simulink model "ScriptDemo"  (R2022b)
settings: configuration reference "TmVcThermal_Configuration_sub" (kept outside this file)
undefined symbols (not defined in the file): aaaa, bbbb, cTmComprCtrl_D_u8HvacFlowTable_db, cTmComprCtrl_D_u8HvacFlowTable_sw, cTmComprCtrl_n_i16ChillCmpIMax, cTmComprCtrl_n_i16ChillCmpIMin, cTmComprCtrl_n_i16ChillCmpIMin666, cTmComprCtrl_n_i16ChillCmpPMax, cTmComprCtrl_n_i16ChillCmpPMin, cTmComprCtrl_n_i16CmpChillCoolRpmKiMax, cTmComprCtrl_n_i16CmpChillCoolRpmKiMin, cTmComprCtrl_n_i16CmpChillCoolRpmKpMax, cTmComprCtrl_n_i16CmpChillCoolRpmKpMin, cTmComprCtrl_n_i16CmpCoolRpmKiMax, cTmComprCtrl_n_i16CmpCoolRpmKiMin, cTmComprCtrl_n_i16CmpCoolRpmKpMax, cTmComprCtrl_n_i16CmpCoolRpmKpMin, cTmComprCtrl_n_i16SM4CmpHeatKiMax, cTmComprCtrl_n_i16SM4CmpHeatKiMin, cTmComprCtrl_n_i16SM4CmpHeatKpMax, cTmComprCtrl_n_i16SM4CmpHeatKpMin, cTmComprCtrl_n_i16SM5CmpHeatKiMax, cTmComprCtrl_n_i16SM5CmpHeatKiMin, cTmComprCtrl_n_i16SM5CmpHeatKpMax, cTmComprCtrl_n_i16SM5CmpHeatKpMin, cTmComprCtrl_n_i16SM6CmpHeatKiMax, cTmComprCtrl_n_i16SM6CmpHeatKiMin, cTmComprCtrl_n_i16SM6CmpHeatKpMax, cTmComprCtrl_n_i16SM6CmpHeatKpMin, cTmComprCtrl_n_u16CmpMaxSpdFanFltLimt, cTmComprCtrl_n_u16CmpMaxSpdLoSidePFltLimt, cTmComprCtrl_n_u16CmpMaxSpdSensorFltLimt, cTmComprCtrl_n_u16CompMinRpm, cTmComprCtrl_n_u16CompRpmIncThres, cTmComprCtrl_t_u16BattCooltFFPeriod, cTmComprCtrl_t_u16BattCooltPIPeriod, cTmComprCtrl_t_u16CmpCoolFFPeriod, cTmComprCtrl_t_u16CmpCoolPIPeriod, cTmComprCtrl_t_u16CoolCmpChillFFPeriod, cTmComprCtrl_t_u16CoolCmpChillPIPeriod, cTmComprCtrl_t_u16SM4CmpHeatFFPeriod, cTmComprCtrl_t_u16SM4CmpHeatPIPeriod, cTmComprCtrl_t_u16SM5CmpHeatFFPeriod, cTmComprCtrl_t_u16SM5CmpHeatPIPeriod, cTmComprCtrl_t_u16SM6CmpHeatFFPeriod, cTmComprCtrl_t_u16SM6CmpHeatPIPeriod, cTmComprCtrl_Te_EvapClearInteg, cTmComprCtrl_Te_i16HpReqTempSaturoffset, cTmComprCtrl_Te_i16SatLpReplaceDiff, cTmComprCtrl_Te_i16SM3BatDiffStartEvapDecOffset, cTmComprCtrl_Te_i16SM3EvapLo, cTmComprCtrl_Te_i16SM3TBatDiffEntEvapDecOffset, cTmComprCtrl_Te_i16SM3TBatDiffEntEvapDecOffsetQuit, cTmComprCtrl_Te_s32ErrCmpChillPIContinueCoolH, cTmComprCtrl_Te_s32ErrCmpChillPIContinueCoolL, cTmComprCtrl_Te_s32ErrCmpPIContinueChillH, cTmComprCtrl_Te_s32ErrCmpPIContinueChillL, cTmComprCtrl_Te_s32ErrCmpPIContinueCoolH, cTmComprCtrl_Te_s32ErrCmpPIContinueCoolL, cTmComprCtrl_Te_s32ErrCmpPIContinueHeatH ... (+398)
libraries: simulink x782, PCMULib x640, simulink_need_slupdate x4
(part 23 of 41)

== system ScriptDemo/Create/createMerge/Before/SM5/SM5_Ki ==
  sTmComprCtrl_D_u8HvacFlowLevel : Inport  OutDataTypeStr=uint8
  sTmSigProces_Te_s32SatLp : Inport  Port=2
  rTmComprCtrl_Te_s32TempError : Inport  Port=3
  Data Type Conversion : DataTypeConversion  OutDataTypeStr=uint16  SaturateOnIntegerOverflow=off  RndMeth=Floor
  Flow2Rpm : Subsystem  mask{BlwHeatLevel_db=cTmComprCtrl_D_u8HvacFlowTable_db, BlwHeatLevel_sw=cTmComprCtrl_D_u8HvacFlowTable_sw, FFBlw1=mTmComprCtrl_n_u16KiSM5CompHeatRpm_Flow1, FFBlw1_Y=mTmComprCtrl_n_u16KiSM5CompHeatRpm_Flow1_Y, FFBlw1_X=mTmComprCtrl_n_u16KiSM5CompHeatRpm_Flow1_X, FFBlw3=mTmComprCtrl_n_u16KiSM5CompHeatRpm_Flow3, FFBlw3_Y=mTmComprCtrl_n_u16KiSM5CompHeatRpm_Flow3_Y, FFBlw3_X=mTmComprCtrl_n_u16KiSM5CompHeatRpm_Flow3_X, FFBlw5=mTmComprCtrl_n_u16KiSM5CompHeatRpm_Flow5, FFBlw5_Y=mTmComprCtrl_n_u16KiSM5CompHeatRpm_Flow5_Y, FFBlw5_X=mTmComprCtrl_n_u16KiSM5CompHeatRpm_Flow5_X, FFBlw7=mTmComprCtrl_n_u16KiSM5CompHeatRpm_Flow7, FFBlw7_Y=mTmComprCtrl_n_u16KiSM5CompHeatRpm_Flow7_Y, FFBlw7_X=mTmComprCtrl_n_u16KiSM5CompHeatRpm_Flow7_X, FFBlw9=mTmComprCtrl_n_u16KiSM5CompHeatRpm_Flow9, FFBlw9_Y=mTmComprCtrl_n_u16KiSM5CompHeatRpm_Flow9_Y, FFBlw9_X=mTmComprCtrl_n_u16KiSM5CompHeatRpm_Flow9_X}
      mask DialogControl ParameterGroupVar Prompt: 参数
  SM5Ki : Outport
  wires:
  Flow2Rpm/1(Flow2Rpm) -> Data Type Conversion/1
  Data Type Conversion/1 -> SM5Ki/1
  sTmComprCtrl_D_u8HvacFlowLevel/1 -> Flow2Rpm/1(md_u8Blw)
  sTmSigProces_Te_s32SatLp/1 -> Flow2Rpm/2(breakpoint1)
  rTmComprCtrl_Te_s32TempError/1 -> Flow2Rpm/3(breakpoint2)

== system ScriptDemo/Create/createMerge/Before/SM5/SM5_Kp ==
  sTmComprCtrl_D_u8HvacFlowLevel : Inport  OutDataTypeStr=uint8
  sTmSigProces_Te_s32SatLp : Inport  Port=2
  rTmComprCtrl_Te_s32TempError : Inport  Port=3
  Data Type Conversion : DataTypeConversion  OutDataTypeStr=uint16  SaturateOnIntegerOverflow=off  RndMeth=Floor
  Flow2Rpm : Subsystem  mask{BlwHeatLevel_db=cTmComprCtrl_D_u8HvacFlowTable_db, BlwHeatLevel_sw=cTmComprCtrl_D_u8HvacFlowTable_sw, FFBlw1=mTmComprCtrl_n_u16KpSM5CompHeatRpm_Flow1, FFBlw1_Y=mTmComprCtrl_n_u16KpSM5CompHeatRpm_Flow1_Y, FFBlw1_X=mTmComprCtrl_n_u16KpSM5CompHeatRpm_Flow1_X, FFBlw3=mTmComprCtrl_n_u16KpSM5CompHeatRpm_Flow3, FFBlw3_Y=mTmComprCtrl_n_u16KpSM5CompHeatRpm_Flow3_Y, FFBlw3_X=mTmComprCtrl_n_u16KpSM5CompHeatRpm_Flow3_X, FFBlw5=mTmComprCtrl_n_u16KpSM5CompHeatRpm_Flow5, FFBlw5_Y=mTmComprCtrl_n_u16KpSM5CompHeatRpm_Flow5_Y, FFBlw5_X=mTmComprCtrl_n_u16KpSM5CompHeatRpm_Flow5_X, FFBlw7=mTmComprCtrl_n_u16KpSM5CompHeatRpm_Flow7, FFBlw7_Y=mTmComprCtrl_n_u16KpSM5CompHeatRpm_Flow7_Y, FFBlw7_X=mTmComprCtrl_n_u16KpSM5CompHeatRpm_Flow7_X, FFBlw9=mTmComprCtrl_n_u16KpSM5CompHeatRpm_Flow9, FFBlw9_Y=mTmComprCtrl_n_u16KpSM5CompHeatRpm_Flow9_Y, FFBlw9_X=mTmComprCtrl_n_u16KpSM5CompHeatRpm_Flow9_X}
      mask DialogControl ParameterGroupVar Prompt: 参数
  SM5Kp : Outport
  wires:
  Flow2Rpm/1(Flow2Rpm) -> Data Type Conversion/1
  Data Type Conversion/1 -> SM5Kp/1
  sTmSigProces_Te_s32SatLp/1 -> Flow2Rpm/2(breakpoint1)
  rTmComprCtrl_Te_s32TempError/1 -> Flow2Rpm/3(breakpoint2)
  sTmComprCtrl_D_u8HvacFlowLevel/1 -> Flow2Rpm/1(md_u8Blw)

== system ScriptDemo/Create/createMerge/Before/SM6/ID26282_SM6FF ==
  note: TODO: 这里需要确认下需求
  sTmComprCtrl_D_u8HvacFlowLevel : Inport  OutDataTypeStr=uint8
  sTmSigProces_Te_s32TempInlet : Inport  Port=2
  sTmSigProces_Te_s32HeatrAirTReqRamp : Inport  Port=3
  Enable : EnablePort
  Flow2Rpm : Subsystem  mask{BlwHeatLevel_db=cTmComprCtrl_D_u8HvacFlowTable_db, BlwHeatLevel_sw=cTmComprCtrl_D_u8HvacFlowTable_sw, FFBlw1=mTmComprCtrl_n_u16FFSM6CompHeatRpm_Flow1, FFBlw1_Y=mTmComprCtrl_n_u16FFSM6CompHeatRpm_Flow1_Y, FFBlw1_X=mTmComprCtrl_n_u16FFSM6CompHeatRpm_Flow1_X, FFBlw3=mTmComprCtrl_n_u16FFSM6CompHeatRpm_Flow3, FFBlw3_Y=mTmComprCtrl_n_u16FFSM6CompHeatRpm_Flow3_Y, FFBlw3_X=mTmComprCtrl_n_u16FFSM6CompHeatRpm_Flow3_X, FFBlw5=mTmComprCtrl_n_u16FFSM6CompHeatRpm_Flow5, FFBlw5_Y=mTmComprCtrl_n_u16FFSM6CompHeatRpm_Flow5_Y, FFBlw5_X=mTmComprCtrl_n_u16FFSM6CompHeatRpm_Flow5_X, FFBlw7=mTmComprCtrl_n_u16FFSM6CompHeatRpm_Flow7, FFBlw7_Y=mTmComprCtrl_n_u16FFSM6CompHeatRpm_Flow7_Y, FFBlw7_X=mTmComprCtrl_n_u16FFSM6CompHeatRpm_Flow7_X, FFBlw9=mTmComprCtrl_n_u16FFSM6CompHeatRpm_Flow9, FFBlw9_Y=mTmComprCtrl_n_u16FFSM6CompHeatRpm_Flow9_Y, FFBlw9_X=mTmComprCtrl_n_u16FFSM6CompHeatRpm_Flow9_X}
      mask DialogControl ParameterGroupVar Prompt: 参数
  SM6FF : Outport
  wires:
  Flow2Rpm/1(Flow2Rpm) -> SM6FF/1
  sTmComprCtrl_D_u8HvacFlowLevel/1 -> Flow2Rpm/1(md_u8Blw)
  sTmSigProces_Te_s32HeatrAirTReqRamp/1 -> Flow2Rpm/3(breakpoint2)
  sTmSigProces_Te_s32TempInlet/1 -> Flow2Rpm/2(breakpoint1)

== system ScriptDemo/Create/createMerge/Before/SM6/ID26284_SM6Error ==
  note: 暖风芯体背风温度目标值∈[0, 80] ℃ 。
  note: 无PTC补热
  note: PTC 补热模式
  sTmSigProces_Te_s32SatHp : Inport
  yTmHvchCtrl_B_HpcPtcEnad : Inport  Port=2
  sTmSigProces_Te_s32HeatrAirTReqRamp : Inport  Port=3
  sTmSigProces_Te_s32HvacHexAirTFilter : Inport  Port=4
  Add2 : Sum
  Constant5 : Constant  Value=cTmComprCtrl_Te_i16HpReqTempSaturoffset
  NegAndPosCheck 4 : Subsystem  AncestorBlock=CustomLib/TempNegAndPosCheck
  NegAndPosCheck 5 : Subsystem  AncestorBlock=CustomLib/TempNegAndPosCheck
  Saturation2 : Saturate  UpperLimit=70  LowerLimit=15
  Switch2 : Switch  Criteria=u2 ~= 0  SaturateOnIntegerOverflow=off  InputSameDT=off
  Terminator : Terminator
  Terminator1 : Terminator
  Unary Minus : UnaryMinus
  rTmComprCtrl_Te_s32TempError : Outport
  wires:
  sTmSigProces_Te_s32SatHp/1 -> NegAndPosCheck 4/2(Acture)
  NegAndPosCheck 5/1(Dvt) -> Switch2/3
  sTmSigProces_Te_s32HeatrAirTReqRamp/1 -> Saturation2/1
  Switch2/1 -> Unary Minus/1
  NegAndPosCheck 5/2(Dvt_PosFlag) -> Terminator/1
  NegAndPosCheck 4/1(Dvt) -> Switch2/1
  Constant5/1 -> Add2/1
  NegAndPosCheck 4/2(Dvt_PosFlag) -> Terminator1/1
  sTmSigProces_Te_s32HvacHexAirTFilter/1 -> NegAndPosCheck 5/2(Acture)
  yTmHvchCtrl_B_HpcPtcEnad/1 -> Switch2/2
  Saturation2/1 -> NegAndPosCheck 5/1(SetPoint), Add2/2
  Add2/1 -> NegAndPosCheck 4/1(SetPoint)
  Unary Minus/1 -> rTmComprCtrl_Te_s32TempError/1

== system ScriptDemo/Create/createMerge/Before/SM6/SM6FFEnable ==
  xTmComprCtrl_B_CompOnReqCompOn : Inport  OutDataTypeStr=boolean
  Compare To Constant2 : simulink/Logic and Bit Operations/Compare To Constant  relop===  const=0  OutDataTypeStr=boolean
  Compare To Constant3 : simulink/Logic and Bit Operations/Compare To Constant  relop===  const=1  OutDataTypeStr=boolean
  Logical Operator3 : Logic  AllPortsSameDT=off  OutDataTypeStr=boolean
  PeriodTrig : Subsystem  mask{CounterLim=cTmComprCtrl_t_u16SM6CmpHeatFFPeriod}
      mask DialogControl ParameterGroupVar Prompt: 参数
  Unit Delay : UnitDelay  SampleTime=-1  HasFrameUpgradeWarning=on
  SM6FFEnable_B_SM6FFEnable : Outport  OutDataTypeStr=boolean
  wires:
  Unit Delay/1 -> Compare To Constant2/1
  [xTmComprCtrl_B_CompOnReqCompOn] -> Compare To Constant3/1, Unit Delay/1
  Compare To Constant2/1 -> Logical Operator3/1
  Logical Operator3/1 -> PeriodTrig/1(Counter_Reset)
  Compare To Constant3/1 -> Logical Operator3/2
  xTmComprCtrl_B_CompOnReqCompOn/1 -> [xTmComprCtrl_B_CompOnReqCompOn]
  PeriodTrig/1(Counter_Trig) -> SM6FFEnable_B_SM6FFEnable/1

== system ScriptDemo/Create/createMerge/Before/SM6/SM6_Ki ==
  sTmComprCtrl_D_u8HvacFlowLevel : Inport  OutDataTypeStr=uint8
  sTmSigProces_Te_s32TempInlet : Inport  Port=2
  rTmComprCtrl_Te_s32TempError : Inport  Port=3
  Flow2Rpm : Subsystem  mask{BlwHeatLevel_db=cTmComprCtrl_D_u8HvacFlowTable_db, BlwHeatLevel_sw=cTmComprCtrl_D_u8HvacFlowTable_sw, FFBlw1=mTmComprCtrl_n_u16KiSM6CompHeatRpm_Flow1, FFBlw1_Y=mTmComprCtrl_n_u16KiSM6CompHeatRpm_Flow1_Y, FFBlw1_X=mTmComprCtrl_n_u16KiSM6CompHeatRpm_Flow1_X, FFBlw3=mTmComprCtrl_n_u16KiSM6CompHeatRpm_Flow3, FFBlw3_Y=mTmComprCtrl_n_u16KiSM6CompHeatRpm_Flow3_Y, FFBlw3_X=mTmComprCtrl_n_u16KiSM6CompHeatRpm_Flow3_X, FFBlw5=mTmComprCtrl_n_u16KiSM6CompHeatRpm_Flow5, FFBlw5_Y=mTmComprCtrl_n_u16KiSM6CompHeatRpm_Flow5_Y, FFBlw5_X=mTmComprCtrl_n_u16KiSM6CompHeatRpm_Flow5_X, FFBlw7=mTmComprCtrl_n_u16KiSM6CompHeatRpm_Flow7, FFBlw7_Y=mTmComprCtrl_n_u16KiSM6CompHeatRpm_Flow7_Y, FFBlw7_X=mTmComprCtrl_n_u16KiSM6CompHeatRpm_Flow7_X, FFBlw9=mTmComprCtrl_n_u16KiSM6CompHeatRpm_Flow9, FFBlw9_Y=mTmComprCtrl_n_u16KiSM6CompHeatRpm_Flow9_Y, FFBlw9_X=mTmComprCtrl_n_u16KiSM6CompHeatRpm_Flow9_X}
      mask DialogControl ParameterGroupVar Prompt: 参数
  SM6Ki : Outport
  wires:
  Flow2Rpm/1(Flow2Rpm) -> SM6Ki/1
  sTmSigProces_Te_s32TempInlet/1 -> Flow2Rpm/2(breakpoint1)
  sTmComprCtrl_D_u8HvacFlowLevel/1 -> Flow2Rpm/1(md_u8Blw)
  rTmComprCtrl_Te_s32TempError/1 -> Flow2Rpm/3(breakpoint2)

== system ScriptDemo/Create/createMerge/Before/SM6/SM6_Kp ==
  sTmComprCtrl_D_u8HvacFlowLevel : Inport  OutDataTypeStr=uint8
  sTmSigProces_Te_s32TempInlet : Inport  Port=2
  rTmComprCtrl_Te_s32TempError : Inport  Port=3
  Flow2Rpm : Subsystem  mask{BlwHeatLevel_db=cTmComprCtrl_D_u8HvacFlowTable_db, BlwHeatLevel_sw=cTmComprCtrl_D_u8HvacFlowTable_sw, FFBlw1=mTmComprCtrl_n_u16KpSM6CompHeatRpm_Flow1, FFBlw1_Y=mTmComprCtrl_n_u16KpSM6CompHeatRpm_Flow1_Y, FFBlw1_X=mTmComprCtrl_n_u16KpSM6CompHeatRpm_Flow1_X, FFBlw3=mTmComprCtrl_n_u16KpSM6CompHeatRpm_Flow3, FFBlw3_Y=mTmComprCtrl_n_u16KpSM6CompHeatRpm_Flow3_Y, FFBlw3_X=mTmComprCtrl_n_u16KpSM6CompHeatRpm_Flow3_X, FFBlw5=mTmComprCtrl_n_u16KpSM6CompHeatRpm_Flow5, FFBlw5_Y=mTmComprCtrl_n_u16KpSM6CompHeatRpm_Flow5_Y, FFBlw5_X=mTmComprCtrl_n_u16KpSM6CompHeatRpm_Flow5_X, FFBlw7=mTmComprCtrl_n_u16KpSM6CompHeatRpm_Flow7, FFBlw7_Y=mTmComprCtrl_n_u16KpSM6CompHeatRpm_Flow7_Y, FFBlw7_X=mTmComprCtrl_n_u16KpSM6CompHeatRpm_Flow7_X, FFBlw9=mTmComprCtrl_n_u16KpSM6CompHeatRpm_Flow9, FFBlw9_Y=mTmComprCtrl_n_u16KpSM6CompHeatRpm_Flow9_Y, FFBlw9_X=mTmComprCtrl_n_u16KpSM6CompHeatRpm_Flow9_X}
      mask DialogControl ParameterGroupVar Prompt: 参数
  SM6Kp : Outport
  wires:
  Flow2Rpm/1(Flow2Rpm) -> SM6Kp/1
  sTmComprCtrl_D_u8HvacFlowLevel/1 -> Flow2Rpm/1(md_u8Blw)
  sTmSigProces_Te_s32TempInlet/1 -> Flow2Rpm/2(breakpoint1)
  rTmComprCtrl_Te_s32TempError/1 -> Flow2Rpm/3(breakpoint2)

== system ScriptDemo/Create/createPorts/createPortsGotoUpdate/After/AllowedPower ==
  note: 压缩机不满足开启条件
  note: 压缩机满足开启条件
  note: 压缩机允许功率
  sTmIn_Pw_s32HvCoolgAllwd : Inport
  xTmComprCtrl_B_CompOnReqCompOn : Inport  Port=2
  Compare To Constant : simulink/Logic and Bit Operations/Compare To Constant  relop=>=  const=6500  OutDataTypeStr=boolean
  Compare To Constant1 : simulink/Logic and Bit Operations/Compare To Constant  relop===  const=6500  OutDataTypeStr=boolean
  Constant2 : Constant  Value=0  OutDataTypeStr=single
  Constant4 : Constant  Value=6500  OutDataTypeStr=single
  Switch1 : Switch  Criteria=u2 ~= 0  SaturateOnIntegerOverflow=off  InputSameDT=off
  Switch3 : Switch  Criteria=u2 ~= 0  Threshold=6500  SaturateOnIntegerOverflow=off  InputSameDT=off
  sTmComprCtrl_Pw_s32ElacCmprMaxState : Outport
  yTmComprCtrl_B_HpcCoolgLimd : Outport  Port=2
  wires:
  sTmIn_Pw_s32HvCoolgAllwd/1 -> Switch3/3, Compare To Constant/1
  Constant2/1 -> Switch1/3
  xTmComprCtrl_B_CompOnReqCompOn/1 -> Switch1/2
  Switch3/1 -> Switch1/1
  Switch1/1 -> Compare To Constant1/1, sTmComprCtrl_Pw_s32ElacCmprMaxState/1
  Constant4/1 -> Switch3/1
  Compare To Constant/1 -> Switch3/2
  Compare To Constant1/1 -> yTmComprCtrl_B_HpcCoolgLimd/1

== system ScriptDemo/Create/createPorts/createPortsGotoUpdate/After1/AllowedPower ==
  note: 压缩机不满足开启条件
  note: 压缩机满足开启条件
  note: 压缩机允许功率
  sTmIn_Pw_s32HvCoolgAllwd : Inport
  xTmComprCtrl_B_CompOnReqCompOn : Inport  Port=2
  Compare To Constant : simulink/Logic and Bit Operations/Compare To Constant  relop=>=  const=6500  OutDataTypeStr=boolean
  Compare To Constant1 : simulink/Logic and Bit Operations/Compare To Constant  relop===  const=6500  OutDataTypeStr=boolean
  Constant2 : Constant  Value=0  OutDataTypeStr=single
  Constant4 : Constant  Value=6500  OutDataTypeStr=single
  Switch1 : Switch  Criteria=u2 ~= 0  SaturateOnIntegerOverflow=off  InputSameDT=off
  Switch3 : Switch  Criteria=u2 ~= 0  Threshold=6500  SaturateOnIntegerOverflow=off  InputSameDT=off
  sTmComprCtrl_Pw_s32ElacCmprMaxState : Outport
  yTmComprCtrl_B_HpcCoolgLimd : Outport  Port=2
  wires:
  sTmIn_Pw_s32HvCoolgAllwd/1 -> Switch3/3, Compare To Constant/1
  Constant2/1 -> Switch1/3
  xTmComprCtrl_B_CompOnReqCompOn/1 -> Switch1/2
  Switch3/1 -> Switch1/1
  Switch1/1 -> Compare To Constant1/1, sTmComprCtrl_Pw_s32ElacCmprMaxState/1
  Constant4/1 -> Switch3/1
  Compare To Constant/1 -> Switch3/2
  Compare To Constant1/1 -> yTmComprCtrl_B_HpcCoolgLimd/1

== system ScriptDemo/Create/createPorts/createPortsGotoUpdate/Before/AllowedPower ==
  note: 压缩机不满足开启条件
  note: 压缩机满足开启条件
  note: 压缩机允许功率
  sTmIn_Pw_s32HvCoolgAllwd : Inport
  xTmComprCtrl_B_CompOnReqCompOn : Inport  Port=2
  Compare To Constant : simulink/Logic and Bit Operations/Compare To Constant  relop=>=  const=6500  OutDataTypeStr=boolean
  Compare To Constant1 : simulink/Logic and Bit Operations/Compare To Constant  relop===  const=6500  OutDataTypeStr=boolean
  Constant2 : Constant  Value=0  OutDataTypeStr=single
  Constant4 : Constant  Value=6500  OutDataTypeStr=single
  Switch1 : Switch  Criteria=u2 ~= 0  SaturateOnIntegerOverflow=off  InputSameDT=off
  Switch3 : Switch  Criteria=u2 ~= 0  Threshold=6500  SaturateOnIntegerOverflow=off  InputSameDT=off
  sTmComprCtrl_Pw_s32ElacCmprMaxState : Outport
  yTmComprCtrl_B_HpcCoolgLimd : Outport  Port=2
  wires:
  sTmIn_Pw_s32HvCoolgAllwd/1 -> Switch3/3, Compare To Constant/1
  Constant2/1 -> Switch1/3
  xTmComprCtrl_B_CompOnReqCompOn/1 -> Switch1/2
  Switch3/1 -> Switch1/1
  Switch1/1 -> Compare To Constant1/1, sTmComprCtrl_Pw_s32ElacCmprMaxState/1
  Constant4/1 -> Switch3/1
  Compare To Constant/1 -> Switch3/2
  Compare To Constant1/1 -> yTmComprCtrl_B_HpcCoolgLimd/1

== system ScriptDemo/Create/createPorts/createPortsGotoUpdateLoop/After/Level3 ==
  sTmIn_Pw_s32HvCoolgAllwd : Inport  OutDataTypeStr=single
  xTmComprCtrl_B_CompOnReqCompOn : Inport  Port=2  OutDataTypeStr=boolean
  xTmComprCtrl_B_AddedSignal : Inport  Port=3  OutDataTypeStr=boolean
  Level2 : Subsystem
  sTmComprCtrl_Pw_s32ElacCmprMaxState : Outport  OutDataTypeStr=single
  yTmComprCtrl_B_HpcCoolgLimd : Outport  Port=2  OutDataTypeStr=boolean
  wires:
  [sTmIn_Pw_s32HvCoolgAllwd] -> Level2/1(sTmIn_Pw_s32HvCoolgAllwd)
  [xTmComprCtrl_B_CompOnReqCompOn] -> Level2/2(xTmComprCtrl_B_CompOnReqCompOn)
  Level2/1(sTmComprCtrl_Pw_s32ElacCmprMaxState) -> [sTmComprCtrl_Pw_s32ElacCmprMaxState]
  Level2/2(yTmComprCtrl_B_HpcCoolgLimd) -> [yTmComprCtrl_B_HpcCoolgLimd]
  sTmIn_Pw_s32HvCoolgAllwd/1 -> [sTmIn_Pw_s32HvCoolgAllwd]
  xTmComprCtrl_B_CompOnReqCompOn/1 -> [xTmComprCtrl_B_CompOnReqCompOn]
  [sTmComprCtrl_Pw_s32ElacCmprMaxState] -> sTmComprCtrl_Pw_s32ElacCmprMaxState/1
  [yTmComprCtrl_B_HpcCoolgLimd] -> yTmComprCtrl_B_HpcCoolgLimd/1
  [xTmComprCtrl_B_AddedSignal] -> Level2/3(xTmComprCtrl_B_AddedSignal)
  xTmComprCtrl_B_AddedSignal/1 -> [xTmComprCtrl_B_AddedSignal]

== system ScriptDemo/Create/createPorts/createPortsGotoUpdateLoop/Before/Level3 ==
  sTmIn_Pw_s32HvCoolgAllwd : Inport  OutDataTypeStr=single
  xTmComprCtrl_B_CompOnReqCompOn : Inport  Port=2  OutDataTypeStr=boolean
  Level2 : Subsystem
  sTmComprCtrl_Pw_s32ElacCmprMaxState : Outport  OutDataTypeStr=single
  yTmComprCtrl_B_HpcCoolgLimd : Outport  Port=2  OutDataTypeStr=boolean
  wires:
  [sTmIn_Pw_s32HvCoolgAllwd] -> Level2/1(sTmIn_Pw_s32HvCoolgAllwd)
  [xTmComprCtrl_B_CompOnReqCompOn] -> Level2/2(xTmComprCtrl_B_CompOnReqCompOn)
  Level2/1(sTmComprCtrl_Pw_s32ElacCmprMaxState) -> [sTmComprCtrl_Pw_s32ElacCmprMaxState]
  Level2/2(yTmComprCtrl_B_HpcCoolgLimd) -> [yTmComprCtrl_B_HpcCoolgLimd]
  sTmIn_Pw_s32HvCoolgAllwd/1 -> [sTmIn_Pw_s32HvCoolgAllwd]
  xTmComprCtrl_B_CompOnReqCompOn/1 -> [xTmComprCtrl_B_CompOnReqCompOn]
  [sTmComprCtrl_Pw_s32ElacCmprMaxState] -> sTmComprCtrl_Pw_s32ElacCmprMaxState/1
  [yTmComprCtrl_B_HpcCoolgLimd] -> yTmComprCtrl_B_HpcCoolgLimd/1

== system ScriptDemo/Create/Model/createModGotoAll/After/TAmbLimit/SM456 ==
  rTmComprCtrl_n_u16CompRpmReqBoundary : Inport  OutDataTypeStr=uint16
  sTmSigProces_Te_s32TAmb : Inport  Port=2  OutDataTypeStr=single
  sTmSigProces_Pw_i16ReqPwrForHeat : Inport  Port=3  OutDataTypeStr=int16
  Enable : EnablePort
  1-D Lookup Table : Lookup_n-D  BreakpointsForDimension1=mTmComprCtrl_n_s32CmpMaxSpdForAmb_Y  BreakpointsForDimension2=mTmComprCtrl_n_s32CmpMaxSpdForAmb_X  BreakpointsForDimension1DataTypeStr=Inherit: Inherit from 'Breakpoint data'  BreakpointsForDimension2DataTypeStr=Inherit: Inherit from 'Breakpoint data'  Table=mTmComprCtrl_n_s32CmpMaxSpdForAmb  TableDataTypeStr=Inherit: Inherit from 'Table data'  ExtrapMethod=Clip  InternalRulePriority=Speed  OutDataTypeStr=Inherit: Inherit via back propagation  RndMeth=Simplest  InputSameDT=off
      settings: InputPortMap=u0,u1
  Relational Operator : RelationalOperator  Operator=>  OutDataTypeStr=boolean  RndMeth=Simplest  InputSameDT=off
  xSM456_B_CmpMaxSpdForAmbFlag : Outport  OutDataTypeStr=boolean
  sSM456_n_u16CompMaxRpm : Outport  Port=2  OutDataTypeStr=uint16
  wires:
  [sTmComprCtrl_n_u16CompMaxRpm] -> Relational Operator/2
  [sTmSigProces_Pw_i16ReqPwrForHeat] -> 1-D Lookup Table/1
  [rTmComprCtrl_n_u16CompRpmReqBoundary] -> Relational Operator/1
  1-D Lookup Table/1 -> [sTmComprCtrl_n_u16CompMaxRpm]
  [sTmSigProces_Te_s32TAmb] -> 1-D Lookup Table/2
  Relational Operator/1 -> [xTmComprCtrl_B_CmpAmbLimtFlag]
  rTmComprCtrl_n_u16CompRpmReqBoundary/1 -> [rTmComprCtrl_n_u16CompRpmReqBoundary]
  sTmSigProces_Te_s32TAmb/1 -> [sTmSigProces_Te_s32TAmb]
  sTmSigProces_Pw_i16ReqPwrForHeat/1 -> [sTmSigProces_Pw_i16ReqPwrForHeat]
  [xTmComprCtrl_B_CmpAmbLimtFlag] -> xSM456_B_CmpMaxSpdForAmbFlag/1
  [sTmComprCtrl_n_u16CompMaxRpm] -> sSM456_n_u16CompMaxRpm/1

== system ScriptDemo/Create/Model/createModGotoAll/After/TAmbLimit/SM456E ==
  Enable : EnablePort
  Constant : Constant  Value=8000  OutDataTypeStr=uint16
  Constant1 : Constant  Value=0  OutDataTypeStr=boolean
  sSM456E_n_u16CompMaxRpm : Outport  OutDataTypeStr=uint16
  xSM456E_B_CmpMaxSpdForAmbFlag : Outport  Port=2  OutDataTypeStr=boolean
  wires:
  Constant/1 -> [sTmComprCtrl_n_u16CompMaxRpm]
  Constant1/1 -> [xTmComprCtrl_B_CmpAmbLimtFlag]
  [sTmComprCtrl_n_u16CompMaxRpm] -> sSM456E_n_u16CompMaxRpm/1
  [xTmComprCtrl_B_CmpAmbLimtFlag] -> xSM456E_B_CmpMaxSpdForAmbFlag/1

== system ScriptDemo/Create/Model/createModGotoAll/Before/TAmbLimit/SM456 ==
  rTmComprCtrl_n_u16CompRpmReqBoundary : Inport  OutDataTypeStr=uint16
  sTmSigProces_Te_s32TAmb : Inport  Port=2  OutDataTypeStr=single
  sTmSigProces_Pw_i16ReqPwrForHeat : Inport  Port=3  OutDataTypeStr=int16
  Enable : EnablePort
  1-D Lookup Table : Lookup_n-D  BreakpointsForDimension1=mTmComprCtrl_n_s32CmpMaxSpdForAmb_Y  BreakpointsForDimension2=mTmComprCtrl_n_s32CmpMaxSpdForAmb_X  BreakpointsForDimension1DataTypeStr=Inherit: Inherit from 'Breakpoint data'  BreakpointsForDimension2DataTypeStr=Inherit: Inherit from 'Breakpoint data'  Table=mTmComprCtrl_n_s32CmpMaxSpdForAmb  TableDataTypeStr=Inherit: Inherit from 'Table data'  ExtrapMethod=Clip  InternalRulePriority=Speed  OutDataTypeStr=Inherit: Inherit via back propagation  RndMeth=Simplest  InputSameDT=off
      settings: InputPortMap=u0,u1
  Relational Operator : RelationalOperator  Operator=>  OutDataTypeStr=boolean  RndMeth=Simplest  InputSameDT=off
  xSM456_B_CmpMaxSpdForAmbFlag : Outport  OutDataTypeStr=boolean
  sSM456_n_u16CompMaxRpm : Outport  Port=2  OutDataTypeStr=uint16
  wires:
  [sTmComprCtrl_n_u16CompMaxRpm] -> Relational Operator/2
  [sTmSigProces_Pw_i16ReqPwrForHeat] -> 1-D Lookup Table/1
  [rTmComprCtrl_n_u16CompRpmReqBoundary] -> Relational Operator/1
  1-D Lookup Table/1 -> [sTmComprCtrl_n_u16CompMaxRpm]
  [sTmSigProces_Te_s32TAmb] -> 1-D Lookup Table/2
  Relational Operator/1 -> [xTmComprCtrl_B_CmpAmbLimtFlag]
  rTmComprCtrl_n_u16CompRpmReqBoundary/1 -> [rTmComprCtrl_n_u16CompRpmReqBoundary]
  sTmSigProces_Te_s32TAmb/1 -> [sTmSigProces_Te_s32TAmb]
  sTmSigProces_Pw_i16ReqPwrForHeat/1 -> [sTmSigProces_Pw_i16ReqPwrForHeat]
  [xTmComprCtrl_B_CmpAmbLimtFlag] -> xSM456_B_CmpMaxSpdForAmbFlag/1
  [sTmComprCtrl_n_u16CompMaxRpm] -> sSM456_n_u16CompMaxRpm/1

== system ScriptDemo/Create/Model/createModGotoAll/Before/TAmbLimit/SM456E ==
  Enable : EnablePort
  Constant : Constant  Value=8000  OutDataTypeStr=uint16
  Constant1 : Constant  Value=0  OutDataTypeStr=boolean
  sSM456E_n_u16CompMaxRpm : Outport  OutDataTypeStr=uint16
  xSM456E_B_CmpMaxSpdForAmbFlag : Outport  Port=2  OutDataTypeStr=boolean
  wires:
  Constant/1 -> [sTmComprCtrl_n_u16CompMaxRpm]
  Constant1/1 -> [xTmComprCtrl_B_CmpAmbLimtFlag]
  [sTmComprCtrl_n_u16CompMaxRpm] -> sSM456E_n_u16CompMaxRpm/1
  [xTmComprCtrl_B_CmpAmbLimtFlag] -> xSM456E_B_CmpMaxSpdForAmbFlag/1

== system ScriptDemo/Create/createMerge/After/ID29332_RpmPI/PIControler/PID_Saturation ==
  note: 0=Not saturated
      | 1=Saturated TOP
      | 2=SaturatedBottom
      | 3=Saturated both (?!?)
  up : Inport
  u : Inport  Port=2
  lo : Inport  Port=3
  Data Type Duplicate : DataTypeDuplicate
  Data Type Propagation : simulink/Signal Attributes/Data Type Propagation  PropDataType=fixdt('double')  IfRefDouble=double  IfRefSingle=single  IsSigned=IsSigned1  NumBitsBase=NumBits1  NumBitsMult=1  NumBitsAdd=0  NumBitsAllowFinal=1:128  PropScaling=[]  ValuesUsedBestPrec=[5 -7]  SlopeBase=Slope1  SlopeMult=1  SlopeAdd=0  BiasBase=Bias1  BiasMult=1  BiasAdd=0
  Gain : Gain  Gain=2  ParamDataTypeStr=uint8  OutDataTypeStr=uint8
  HitLowerLimit : RelationalOperator  DisableCoverage=on  Operator=<  OutDataTypeStr=boolean  InputSameDT=off
  HitUpperLimit : RelationalOperator  DisableCoverage=on  Operator=>  OutDataTypeStr=boolean  InputSameDT=off
  Sum : Sum  Inputs=+|+  AccumDataTypeStr=uint8  OutDataTypeStr=uint8
  Switch : Switch  Criteria=u2 ~= 0  OutDataTypeStr=Inherit: Inherit via back propagation  RndMeth=Nearest  ZeroCross=off  InputSameDT=off
  Switch2 : Switch  Criteria=u2 ~= 0  OutMin=OutMin  OutMax=OutMax  RndMeth=Nearest  ZeroCross=off  InputSameDT=off
  y : Outport  OutMin=OutMin  OutMax=OutMax  VectorParamsAs1DForOutWhenUnconnected=off
  N_SaturationState : Outport  Port=2  OutMin=OutMin  OutMax=OutMax  OutDataTypeStr=uint8  VectorParamsAs1DForOutWhenUnconnected=off
  wires:
  Sum/1 -> N_SaturationState/1
  Gain/1 -> Sum/2
  up/1 -> Switch2/1, HitUpperLimit/2
  u/1 -> Data Type Propagation/2, Data Type Propagation/1, HitUpperLimit/1, Switch/3, HitLowerLimit/1
  lo/1 -> Switch/1, HitLowerLimit/2
  Switch/1 -> Data Type Duplicate/2, Switch2/3, Data Type Propagation/3
  Switch2/1 -> Data Type Duplicate/1, y/1
  HitUpperLimit/1 -> Sum/1, Switch2/2
  HitLowerLimit/1 -> Gain/1, Switch/2

== system ScriptDemo/Create/createMerge/After/ID29332_RpmPI/PIControler/SaturationAndDeadband ==
  note: 0=Not saturated
  note: 1=Saturated TOP
  note: 2=SaturatedBottom
  N_SaturationState : Inport
  rTmComprCtrl_Te_s32DeadBand : Inport  Port=2  OutDataTypeStr=single
  rTmComprCtrl_Te_s32LowErrStop : Inport  Port=3  OutDataTypeStr=single
  rTmComprCtrl_Te_s32TempError : Inport  Port=4  OutDataTypeStr=single
  rTmComprCtrl_Te_s32UpErrStop : Inport  Port=5  OutDataTypeStr=single
  xTmComprCtrl_B_ReduceRpm : Inport  Port=6  OutDataTypeStr=boolean
  Abs : Abs  SaturateOnIntegerOverflow=off
  Constant{,2..5} (5 alike) : Constant  Value=0  OutDataTypeStr=Inherit: Inherit via back propagation  SampleTime=-1
  Constant13 : Constant  Value=0  OutDataTypeStr=single
  DB : Switch  Criteria=u2 ~= 0  Threshold=0.5
  ErrorLargerThanDeadband : RelationalOperator  Operator=>  OutDataTypeStr=boolean  ZeroCross=off
  Multiport Switch : MultiPortSwitch  DataPortOrder=Zero-based contiguous  DiagnosticForDefault=None  zeroidx=on  SaturateOnIntegerOverflow=off  InputSameDT=off
  Relay : PCMULib/Standard/Relation&Logic/Relay
      settings: SourceProductName=PCMULib
  Relay2 : PCMULib/Standard/Relation&Logic/Relay
      settings: SourceProductName=PCMULib
  Switch1 : Switch  Criteria=u2 ~= 0  SaturateOnIntegerOverflow=off  InputSameDT=off
  Switch2 : Switch  Criteria=u2 ~= 0  SaturateOnIntegerOverflow=off  InputSameDT=off
  Switch3 : Switch  Criteria=u2 ~= 0  SaturateOnIntegerOverflow=off  InputSameDT=off
  rSaturationAndDeadband_Te_s32TempErrorOut : Outport  OutDataTypeStr=single
  wires:
  [rTmComprCtrl_Te_s32TempError] -> Abs/1, DB/1
  [rTmComprCtrl_Te_s32DeadBand] -> ErrorLargerThanDeadband/2
  Constant/1 -> DB/3
  [N_SaturationState] -> Multiport Switch/1
  ErrorLargerThanDeadband/1 -> DB/2
  Abs/1 -> ErrorLargerThanDeadband/1
  DB/1 -> [rTmComprCtrl_Te_s32TempErrorRaw]
  [rTmComprCtrl_Te_s32TempErrorRaw] -> Multiport Switch/2
  [rTmComprCtrl_Te_s32UpErrStop] -> Relay/2
  [rTmComprCtrl_Te_s32TempErrorRaw] -> Relay/1
  Constant2/1 -> Relay/3
  Relay/1 -> Switch2/2
  Constant3/1 -> Switch2/1
  [rTmComprCtrl_Te_s32TempErrorRaw] -> Switch2/3
  [rTmComprCtrl_Te_s32TempErrorRaw] -> Relay2/1
  Constant4/1 -> Relay2/2
  [rTmComprCtrl_Te_s32LowErrStop] -> Relay2/3
  Relay2/1 -> Switch3/2
  [rTmComprCtrl_Te_s32TempErrorRaw] -> Switch3/1
  Constant5/1 -> Switch3/3
  Switch2/1 -> Multiport Switch/3
  Switch3/1 -> Multiport Switch/4
  N_SaturationState/1 -> [N_SaturationState]
  rTmComprCtrl_Te_s32DeadBand/1 -> [rTmComprCtrl_Te_s32DeadBand]
  rTmComprCtrl_Te_s32LowErrStop/1 -> [rTmComprCtrl_Te_s32LowErrStop]
  rTmComprCtrl_Te_s32TempError/1 -> [rTmComprCtrl_Te_s32TempError]
  rTmComprCtrl_Te_s32UpErrStop/1 -> [rTmComprCtrl_Te_s32UpErrStop]
  [rTmComprCtrl_Te_s32TempErrorOut] -> rSaturationAndDeadband_Te_s32TempErrorOut/1
  [xTmComprCtrl_B_ReduceRpm] -> Switch1/2
  Constant13/1 -> Switch1/1
  Multiport Switch/1 -> Switch1/3
  Switch1/1 -> [rTmComprCtrl_Te_s32TempErrorOut]
  xTmComprCtrl_B_ReduceRpm/1 -> [xTmComprCtrl_B_ReduceRpm]

== system ScriptDemo/Create/createMerge/After/SM1SM21/ID26247_SM1Error/NegAndPosCheck  ==
  SetPoint : Inport
  Acture : Inport  Port=2
  Compare To Constant : simulink/Logic and Bit Operations/Compare To Constant  relop=>=  const=0  OutDataTypeStr=boolean
  Data Type Conversion : DataTypeConversion  SaturateOnIntegerOverflow=off  RndMeth=Floor
  Data Type Conversion1 : DataTypeConversion  SaturateOnIntegerOverflow=off  RndMeth=Floor
  Data Type Conversion2 : DataTypeConversion  SaturateOnIntegerOverflow=off  RndMeth=Floor
  Sum : Sum  Inputs=|-+  OutDataTypeStr=Inherit: Same as first input
  Dvt : Outport  VectorParamsAs1DForOutWhenUnconnected=off
  Dvt_PosFlag : Outport  Port=2  VectorParamsAs1DForOutWhenUnconnected=off
  wires:
  SetPoint/1 -> Data Type Conversion/1
  Acture/1 -> Data Type Conversion1/1
  Sum/1 -> Data Type Conversion2/1
  Compare To Constant/1 -> Dvt_PosFlag/1
  Data Type Conversion/1 -> Sum/1
  Data Type Conversion1/1 -> Sum/2
  Data Type Conversion2/1 -> Compare To Constant/1, Dvt/1

== system ScriptDemo/Create/createMerge/After/SM1SM21/SM1FFEnable/BevvFFPeriod ==
  Counter_Reset : Inport
  Add : Sum
  Add1 : Sum  Inputs=+-
  Constant : Constant  Value=CounterLim
  Constant1 : Constant  Value=cTmSwArch_t_s32SampleTime
      settings: AttributesFormatString=%<Value>
  Constant2 : Constant  Value=0  OutDataTypeStr=single
  Constant50 : Constant  Value=cTmSwArch_t_s32SampleTime
      settings: AttributesFormatString=%<Value>
  Logical Operator : Logic  Operator=OR  AllPortsSameDT=off  OutDataTypeStr=boolean
  Relational Operator : RelationalOperator  OutDataTypeStr=boolean  RndMeth=Simplest  InputSameDT=off
  Switch : Switch  Criteria=u2 ~= 0  SaturateOnIntegerOverflow=off  InputSameDT=off
  Switch1 : Switch  Criteria=u2 ~= 0  SaturateOnIntegerOverflow=off  InputSameDT=off
  Unit Delay : UnitDelay  SampleTime=-1  HasFrameUpgradeWarning=on
  Unit Delay1 : UnitDelay  SampleTime=-1  HasFrameUpgradeWarning=on
  Counter_Trig : Outport
  wires:
  Relational Operator/1 -> Unit Delay1/1, Counter_Trig/1
  [CounterLim] -> Relational Operator/2
  Add/1 -> Unit Delay/1, Relational Operator/1
  Unit Delay/1 -> Switch/3
  Switch/1 -> Add/2
  Constant1/1 -> Add/1
  Logical Operator/1 -> Switch/2
  Counter_Reset/1 -> Switch1/2, Logical Operator/1
  Unit Delay1/1 -> Logical Operator/2
  Constant2/1 -> Switch1/3
  Switch1/1 -> Switch/1
  Add1/1 -> Switch1/1
  Constant50/1 -> Add1/2
  Constant/1 -> [CounterLim]
  [CounterLim] -> Add1/1

== system ScriptDemo/Create/createMerge/After/SM1SM21/SM1_Ki/tableChoose ==
  note: 快充
  note: 非快充，超充
  note: 电池有主动制冷需求
  note: 电池非正常制冷
  note: 超充
  note: 电池有主动制冷需求
  sTmSigProces_D_u8BattThermReq : Inport
  sTmIn_D_u8DCChrgSt : Inport  Port=2
  tab1 : Inport  Port=3
  tab2 : Inport  Port=4
  tab3 : Inport  Port=5
  Compare To Constant : simulink/Logic and Bit Operations/Compare To Constant  relop===  const=2  OutDataTypeStr=boolean
  Compare To Constant1 : simulink/Logic and Bit Operations/Compare To Constant  relop===  const=12  OutDataTypeStr=boolean
  Compare To Constant2 : simulink/Logic and Bit Operations/Compare To Constant  relop===  const=5  OutDataTypeStr=boolean
  Switch2 : Switch  Criteria=u2 ~= 0  SaturateOnIntegerOverflow=off  InputSameDT=off
  Switch4 : Switch  Criteria=u2 ~= 0  SaturateOnIntegerOverflow=off  InputSameDT=off
  Switch5 : Switch  Criteria=u2 ~= 0  SaturateOnIntegerOverflow=off  InputSameDT=off
  电池无主动制冷需求 : Constant  Value=0  OutDataTypeStr=uint16
  out : Outport  OutDataTypeStr=uint16
  wires:
  Compare To Constant1/1 -> Switch5/2
  tab1/1 -> Switch5/3
  tab3/1 -> Switch5/1
  tab2/1 -> Switch4/1
  sTmIn_D_u8DCChrgSt/1 -> Compare To Constant/1, Compare To Constant1/1
  Switch5/1 -> Switch4/3
  sTmSigProces_D_u8BattThermReq/1 -> Compare To Constant2/1
  Compare To Constant2/1 -> Switch2/2
  电池无主动制冷需求/1 -> Switch2/3
  Switch2/1 -> out/1
  Switch4/1 -> Switch2/1
  Compare To Constant/1 -> Switch4/2

== system ScriptDemo/Create/createMerge/After/SM1SM21/SM1_Kp/tableChoose ==
  note: 快充
  note: 非快充，超充
  note: 电池有主动制冷需求
  note: 电池非正常制冷
  note: 超充
  note: 电池有主动制冷需求
  sTmSigProces_D_u8BattThermReq : Inport
  sTmIn_D_u8DCChrgSt : Inport  Port=2
  tab1 : Inport  Port=3
  tab2 : Inport  Port=4
  tab3 : Inport  Port=5
  Compare To Constant : simulink/Logic and Bit Operations/Compare To Constant  relop===  const=2  OutDataTypeStr=boolean
  Compare To Constant1 : simulink/Logic and Bit Operations/Compare To Constant  relop===  const=12  OutDataTypeStr=boolean
  Compare To Constant2 : simulink/Logic and Bit Operations/Compare To Constant  relop===  const=5  OutDataTypeStr=boolean
  Switch2 : Switch  Criteria=u2 ~= 0  SaturateOnIntegerOverflow=off  InputSameDT=off
  Switch4 : Switch  Criteria=u2 ~= 0  SaturateOnIntegerOverflow=off  InputSameDT=off
  Switch5 : Switch  Criteria=u2 ~= 0  SaturateOnIntegerOverflow=off  InputSameDT=off
  电池无主动制冷需求 : Constant  Value=0  OutDataTypeStr=uint16
  out : Outport
  wires:
  Compare To Constant1/1 -> Switch5/2
  tab1/1 -> Switch5/3
  tab3/1 -> Switch5/1
  tab2/1 -> Switch4/1
  sTmIn_D_u8DCChrgSt/1 -> Compare To Constant/1, Compare To Constant1/1
  Switch5/1 -> Switch4/3
  sTmSigProces_D_u8BattThermReq/1 -> Compare To Constant2/1
  Compare To Constant2/1 -> Switch2/2
  电池无主动制冷需求/1 -> Switch2/3
  Switch2/1 -> out/1
  Switch4/1 -> Switch2/1
  Compare To Constant/1 -> Switch4/2

== system ScriptDemo/Create/createMerge/After/SM2SM22/ID26239_SM2Error/NegAndPosCheck 1 ==
  SetPoint : Inport
  Acture : Inport  Port=2
  Compare To Constant : simulink/Logic and Bit Operations/Compare To Constant  relop=>=  const=0  OutDataTypeStr=boolean
  Data Type Conversion : DataTypeConversion  SaturateOnIntegerOverflow=off  RndMeth=Floor
  Data Type Conversion1 : DataTypeConversion  SaturateOnIntegerOverflow=off  RndMeth=Floor
  Data Type Conversion2 : DataTypeConversion  SaturateOnIntegerOverflow=off  RndMeth=Floor
  Sum : Sum  Inputs=|-+  OutDataTypeStr=Inherit: Same as first input
  Dvt : Outport  VectorParamsAs1DForOutWhenUnconnected=off
  Dvt_PosFlag : Outport  Port=2  VectorParamsAs1DForOutWhenUnconnected=off
  wires:
  Data Type Conversion2/1 -> Dvt/1, Compare To Constant/1
  Data Type Conversion1/1 -> Sum/2
  Data Type Conversion/1 -> Sum/1
  Compare To Constant/1 -> Dvt_PosFlag/1
  Sum/1 -> Data Type Conversion2/1
  Acture/1 -> Data Type Conversion1/1
  SetPoint/1 -> Data Type Conversion/1

== system ScriptDemo/Create/createMerge/After/SM2SM22/ID26267_SM2FF/Flow2RpmOsa ==
  md_u8Blw : Inport
  breakpoint1 : Inport  Port=2
  breakpoint2 : Inport  Port=3
  2-D Lookup Table5 : Lookup_n-D  BreakpointsForDimension1=FFBlw1_Y  BreakpointsForDimension2=FFBlw1_X  BreakpointsForDimension1DataTypeStr=Inherit: Inherit from 'Breakpoint data'  BreakpointsForDimension2DataTypeStr=Inherit: Inherit from 'Breakpoint data'  Table=FFBlw1  TableDataTypeStr=Inherit: Inherit from 'Table data'  ExtrapMethod=Clip  InternalRulePriority=Speed  OutDataTypeStr=Inherit: Inherit from 'Table data'  RndMeth=Simplest
      settings: InputPortMap=u0,u1
  2-D Lookup Table6 : Lookup_n-D  BreakpointsForDimension1=FFBlw3_Y  BreakpointsForDimension2=FFBlw3_X  BreakpointsForDimension1DataTypeStr=Inherit: Inherit from 'Breakpoint data'  BreakpointsForDimension2DataTypeStr=Inherit: Inherit from 'Breakpoint data'  Table=FFBlw3  TableDataTypeStr=Inherit: Inherit from 'Table data'  ExtrapMethod=Clip  InternalRulePriority=Speed  OutDataTypeStr=Inherit: Inherit from 'Table data'  RndMeth=Simplest
      settings: InputPortMap=u0,u1
  2-D Lookup Table7 : Lookup_n-D  BreakpointsForDimension1=FFBlw5_Y  BreakpointsForDimension2=FFBlw5_X  BreakpointsForDimension1DataTypeStr=Inherit: Inherit from 'Breakpoint data'  BreakpointsForDimension2DataTypeStr=Inherit: Inherit from 'Breakpoint data'  Table=FFBlw5  TableDataTypeStr=Inherit: Inherit from 'Table data'  ExtrapMethod=Clip  InternalRulePriority=Speed  OutDataTypeStr=Inherit: Inherit from 'Table data'  RndMeth=Simplest
      settings: InputPortMap=u0,u1
  2-D Lookup Table8 : Lookup_n-D  BreakpointsForDimension1=FFBlw7_Y  BreakpointsForDimension2=FFBlw7_X  BreakpointsForDimension1DataTypeStr=Inherit: Inherit from 'Breakpoint data'  BreakpointsForDimension2DataTypeStr=Inherit: Inherit from 'Breakpoint data'  Table=FFBlw7  TableDataTypeStr=Inherit: Inherit from 'Table data'  ExtrapMethod=Clip  InternalRulePriority=Speed  OutDataTypeStr=Inherit: Inherit from 'Table data'  RndMeth=Simplest
      settings: InputPortMap=u0,u1
  2-D Lookup Table9 : Lookup_n-D  BreakpointsForDimension1=FFBlw9_Y  BreakpointsForDimension2=FFBlw9_X  BreakpointsForDimension1DataTypeStr=Inherit: Inherit from 'Breakpoint data'  BreakpointsForDimension2DataTypeStr=Inherit: Inherit from 'Breakpoint data'  Table=FFBlw9  TableDataTypeStr=Inherit: Inherit from 'Table data'  ExtrapMethod=Clip  InternalRulePriority=Speed  OutDataTypeStr=Inherit: Inherit from 'Table data'  RndMeth=Simplest
      settings: InputPortMap=u0,u1
  Add{2..6} (5 alike) : Sum  Inputs=+-  OutDataTypeStr=int16
  Add7 : Sum  Inputs=+++++
  Constant{,1..4} (5 alike) : Constant  Value=0.1  OutDataTypeStr=single
  Constant5 : Constant  Value=10  OutDataTypeStr=int16
  Constant6 : Constant  Value=20  OutDataTypeStr=int16
  Constant7 : Constant  Value=30  OutDataTypeStr=int16
  Constant8 : Constant  Value=40  OutDataTypeStr=int16
  Constant9 : Constant  Value=50  OutDataTypeStr=int16
  Data Type Conversion : DataTypeConversion  OutDataTypeStr=uint16  SaturateOnIntegerOverflow=off  RndMeth=Floor
  Data Type Conversion1 : DataTypeConversion  OutDataTypeStr=int16  SaturateOnIntegerOverflow=off  RndMeth=Floor
  Product{,1..9} (10 alike) : Product  OutDataTypeStr=single
  Subsystem1 : Subsystem
  Subsystem2 : Subsystem
  Subsystem3 : Subsystem
  Subsystem4 : Subsystem
  Subsystem5 : Subsystem
  XCP : Subsystem
  Flow2Rpm : Outport
  wires:
  Subsystem1/1(Out1) -> Product/2
  Product2/1 -> Product7/2
  [breakpoint2] -> 2-D Lookup Table5/2
  Product4/1 -> Product9/2
  Product9/1 -> Add7/5
  [breakpoint1] -> 2-D Lookup Table7/1
  Constant9/1 -> Add6/1
  [breakpoint1] -> 2-D Lookup Table9/1
  [breakpoint1] -> 2-D Lookup Table5/1
  [breakpoint1] -> 2-D Lookup Table6/1
  Product5/1 -> Add7/1
  2-D Lookup Table7/1 -> Product2/1
  Data Type Conversion1/1 -> Add4/2, Add6/2, Add5/2, Add3/2, Add2/2
  [breakpoint2] -> 2-D Lookup Table8/2
  Product/1 -> Product5/2
  Subsystem5/1(Out1) -> Product4/2
  [breakpoint2] -> 2-D Lookup Table7/2
  Subsystem2/1(Out1) -> Product1/2
  Constant8/1 -> Add5/1
  Product8/1 -> Add7/4
  Constant7/1 -> Add4/1
  Add4/1 -> Subsystem3/1(In1)
  Subsystem3/1(Out1) -> Product2/2
  Subsystem4/1(Out1) -> Product3/2
  Product1/1 -> Product6/2
  Add2/1 -> Subsystem1/1(In1)
  [breakpoint1] -> 2-D Lookup Table8/1
  [breakpoint2] -> 2-D Lookup Table6/2
  2-D Lookup Table5/1 -> Product/1
  Constant5/1 -> Add2/1
  2-D Lookup Table8/1 -> Product3/1
  Constant6/1 -> Add3/1
  Add6/1 -> Subsystem5/1(In1)
  Add5/1 -> Subsystem4/1(In1)
  Product3/1 -> Product8/2
  [breakpoint2] -> 2-D Lookup Table9/2
  Add3/1 -> Subsystem2/1(In1)
  Add7/1 -> Data Type Conversion/1
  2-D Lookup Table6/1 -> Product1/1
  Product7/1 -> Add7/3
  2-D Lookup Table9/1 -> Product4/1
  Product6/1 -> Add7/2
  breakpoint1/1 -> [breakpoint1]
  breakpoint2/1 -> [breakpoint2]
  XCP/1(Out1) -> Data Type Conversion1/1
  Constant/1 -> Product5/1
  Constant1/1 -> Product6/1
  Constant2/1 -> Product7/1
  Constant3/1 -> Product8/1
  Constant4/1 -> Product9/1
  md_u8Blw/1 -> XCP/1(md_u8Blw)
  Data Type Conversion/1 -> Flow2Rpm/1

== system ScriptDemo/Create/createMerge/After/SM2SM22/ID26267_SM2FF/Flow2RpmOsa1 ==
  md_u8Blw : Inport
  breakpoint1 : Inport  Port=2
  breakpoint2 : Inport  Port=3
  2-D Lookup Table5 : Lookup_n-D  BreakpointsForDimension1=FFBlw1_Y  BreakpointsForDimension2=FFBlw1_X  BreakpointsForDimension1DataTypeStr=Inherit: Inherit from 'Breakpoint data'  BreakpointsForDimension2DataTypeStr=Inherit: Inherit from 'Breakpoint data'  Table=FFBlw1  TableDataTypeStr=Inherit: Inherit from 'Table data'  ExtrapMethod=Clip  InternalRulePriority=Speed  OutDataTypeStr=Inherit: Inherit from 'Table data'  RndMeth=Simplest
      settings: InputPortMap=u0,u1
  2-D Lookup Table6 : Lookup_n-D  BreakpointsForDimension1=FFBlw3_Y  BreakpointsForDimension2=FFBlw3_X  BreakpointsForDimension1DataTypeStr=Inherit: Inherit from 'Breakpoint data'  BreakpointsForDimension2DataTypeStr=Inherit: Inherit from 'Breakpoint data'  Table=FFBlw3  TableDataTypeStr=Inherit: Inherit from 'Table data'  ExtrapMethod=Clip  InternalRulePriority=Speed  OutDataTypeStr=Inherit: Inherit from 'Table data'  RndMeth=Simplest
      settings: InputPortMap=u0,u1
  2-D Lookup Table7 : Lookup_n-D  BreakpointsForDimension1=FFBlw5_Y  BreakpointsForDimension2=FFBlw5_X  BreakpointsForDimension1DataTypeStr=Inherit: Inherit from 'Breakpoint data'  BreakpointsForDimension2DataTypeStr=Inherit: Inherit from 'Breakpoint data'  Table=FFBlw5  TableDataTypeStr=Inherit: Inherit from 'Table data'  ExtrapMethod=Clip  InternalRulePriority=Speed  OutDataTypeStr=Inherit: Inherit from 'Table data'  RndMeth=Simplest
      settings: InputPortMap=u0,u1
  2-D Lookup Table8 : Lookup_n-D  BreakpointsForDimension1=FFBlw7_Y  BreakpointsForDimension2=FFBlw7_X  BreakpointsForDimension1DataTypeStr=Inherit: Inherit from 'Breakpoint data'  BreakpointsForDimension2DataTypeStr=Inherit: Inherit from 'Breakpoint data'  Table=FFBlw7  TableDataTypeStr=Inherit: Inherit from 'Table data'  ExtrapMethod=Clip  InternalRulePriority=Speed  OutDataTypeStr=Inherit: Inherit from 'Table data'  RndMeth=Simplest
      settings: InputPortMap=u0,u1
  2-D Lookup Table9 : Lookup_n-D  BreakpointsForDimension1=FFBlw9_Y  BreakpointsForDimension2=FFBlw9_X  BreakpointsForDimension1DataTypeStr=Inherit: Inherit from 'Breakpoint data'  BreakpointsForDimension2DataTypeStr=Inherit: Inherit from 'Breakpoint data'  Table=FFBlw9  TableDataTypeStr=Inherit: Inherit from 'Table data'  ExtrapMethod=Clip  InternalRulePriority=Speed  OutDataTypeStr=Inherit: Inherit from 'Table data'  RndMeth=Simplest
      settings: InputPortMap=u0,u1
  Add{2..6} (5 alike) : Sum  Inputs=+-  OutDataTypeStr=int16
  Add7 : Sum  Inputs=+++++
  Constant{,1..4} (5 alike) : Constant  Value=0.1  OutDataTypeStr=single
  Constant5 : Constant  Value=10  OutDataTypeStr=int16
  Constant6 : Constant  Value=20  OutDataTypeStr=int16
  Constant7 : Constant  Value=30  OutDataTypeStr=int16
  Constant8 : Constant  Value=40  OutDataTypeStr=int16
  Constant9 : Constant  Value=50  OutDataTypeStr=int16
  Data Type Conversion : DataTypeConversion  OutDataTypeStr=uint16  SaturateOnIntegerOverflow=off  RndMeth=Floor
  Data Type Conversion1 : DataTypeConversion  OutDataTypeStr=int16  SaturateOnIntegerOverflow=off  RndMeth=Floor
  Product{,1..9} (10 alike) : Product  OutDataTypeStr=single
  Subsystem1 : Subsystem
  Subsystem2 : Subsystem
  Subsystem3 : Subsystem
  Subsystem4 : Subsystem
  Subsystem5 : Subsystem
  XCP : Subsystem
  Flow2Rpm : Outport
  wires:
  Subsystem1/1(Out1) -> Product/2
  Product2/1 -> Product7/2
  [breakpoint2] -> 2-D Lookup Table5/2
  Product4/1 -> Product9/2
  Product9/1 -> Add7/5
  [breakpoint1] -> 2-D Lookup Table7/1
  Constant9/1 -> Add6/1
  [breakpoint1] -> 2-D Lookup Table9/1
  [breakpoint1] -> 2-D Lookup Table5/1
  [breakpoint1] -> 2-D Lookup Table6/1
  Product5/1 -> Add7/1
  2-D Lookup Table7/1 -> Product2/1
  Data Type Conversion1/1 -> Add4/2, Add6/2, Add5/2, Add3/2, Add2/2
  [breakpoint2] -> 2-D Lookup Table8/2
  Product/1 -> Product5/2
  Subsystem5/1(Out1) -> Product4/2
  [breakpoint2] -> 2-D Lookup Table7/2
  Subsystem2/1(Out1) -> Product1/2
  Constant8/1 -> Add5/1
  Product8/1 -> Add7/4
  Constant7/1 -> Add4/1
  Add4/1 -> Subsystem3/1(In1)
  Subsystem3/1(Out1) -> Product2/2
  Subsystem4/1(Out1) -> Product3/2
  Product1/1 -> Product6/2
  Add2/1 -> Subsystem1/1(In1)
  [breakpoint1] -> 2-D Lookup Table8/1
  [breakpoint2] -> 2-D Lookup Table6/2
  2-D Lookup Table5/1 -> Product/1
  Constant5/1 -> Add2/1
  2-D Lookup Table8/1 -> Product3/1
  Constant6/1 -> Add3/1
  Add6/1 -> Subsystem5/1(In1)
  Add5/1 -> Subsystem4/1(In1)
  Product3/1 -> Product8/2
  [breakpoint2] -> 2-D Lookup Table9/2
  Add3/1 -> Subsystem2/1(In1)
  Add7/1 -> Data Type Conversion/1
  2-D Lookup Table6/1 -> Product1/1
  Product7/1 -> Add7/3
  2-D Lookup Table9/1 -> Product4/1
  Product6/1 -> Add7/2
  breakpoint1/1 -> [breakpoint1]
  breakpoint2/1 -> [breakpoint2]
  XCP/1(Out1) -> Data Type Conversion1/1
  Constant/1 -> Product5/1
  Constant1/1 -> Product6/1
  Constant2/1 -> Product7/1
  Constant3/1 -> Product8/1
  Constant4/1 -> Product9/1
  md_u8Blw/1 -> XCP/1(md_u8Blw)
  Data Type Conversion/1 -> Flow2Rpm/1

== system ScriptDemo/Create/createMerge/After/SM2SM22/ID26267_SM2FF/Flow2RpmRec ==
  md_u8Blw : Inport
  breakpoint1 : Inport  Port=2
  breakpoint2 : Inport  Port=3
  2-D Lookup Table5 : Lookup_n-D  BreakpointsForDimension1=FFBlw1_Y  BreakpointsForDimension2=FFBlw1_X  BreakpointsForDimension1DataTypeStr=Inherit: Inherit from 'Breakpoint data'  BreakpointsForDimension2DataTypeStr=Inherit: Inherit from 'Breakpoint data'  Table=FFBlw1  TableDataTypeStr=Inherit: Inherit from 'Table data'  ExtrapMethod=Clip  InternalRulePriority=Speed  OutDataTypeStr=Inherit: Inherit from 'Table data'  RndMeth=Simplest
      settings: InputPortMap=u0,u1
  2-D Lookup Table6 : Lookup_n-D  BreakpointsForDimension1=FFBlw3_Y  BreakpointsForDimension2=FFBlw3_X  BreakpointsForDimension1DataTypeStr=Inherit: Inherit from 'Breakpoint data'  BreakpointsForDimension2DataTypeStr=Inherit: Inherit from 'Breakpoint data'  Table=FFBlw3  TableDataTypeStr=Inherit: Inherit from 'Table data'  ExtrapMethod=Clip  InternalRulePriority=Speed  OutDataTypeStr=Inherit: Inherit from 'Table data'  RndMeth=Simplest
      settings: InputPortMap=u0,u1
  2-D Lookup Table7 : Lookup_n-D  BreakpointsForDimension1=FFBlw5_Y  BreakpointsForDimension2=FFBlw5_X  BreakpointsForDimension1DataTypeStr=Inherit: Inherit from 'Breakpoint data'  BreakpointsForDimension2DataTypeStr=Inherit: Inherit from 'Breakpoint data'  Table=FFBlw5  TableDataTypeStr=Inherit: Inherit from 'Table data'  ExtrapMethod=Clip  InternalRulePriority=Speed  OutDataTypeStr=Inherit: Inherit from 'Table data'  RndMeth=Simplest
      settings: InputPortMap=u0,u1
  2-D Lookup Table8 : Lookup_n-D  BreakpointsForDimension1=FFBlw7_Y  BreakpointsForDimension2=FFBlw7_X  BreakpointsForDimension1DataTypeStr=Inherit: Inherit from 'Breakpoint data'  BreakpointsForDimension2DataTypeStr=Inherit: Inherit from 'Breakpoint data'  Table=FFBlw7  TableDataTypeStr=Inherit: Inherit from 'Table data'  ExtrapMethod=Clip  InternalRulePriority=Speed  OutDataTypeStr=Inherit: Inherit from 'Table data'  RndMeth=Simplest
      settings: InputPortMap=u0,u1
  2-D Lookup Table9 : Lookup_n-D  BreakpointsForDimension1=FFBlw9_Y  BreakpointsForDimension2=FFBlw9_X  BreakpointsForDimension1DataTypeStr=Inherit: Inherit from 'Breakpoint data'  BreakpointsForDimension2DataTypeStr=Inherit: Inherit from 'Breakpoint data'  Table=FFBlw9  TableDataTypeStr=Inherit: Inherit from 'Table data'  ExtrapMethod=Clip  InternalRulePriority=Speed  OutDataTypeStr=Inherit: Inherit from 'Table data'  RndMeth=Simplest
      settings: InputPortMap=u0,u1
  Add{2..6} (5 alike) : Sum  Inputs=+-  OutDataTypeStr=int16
  Add7 : Sum  Inputs=+++++
  Constant{,1..4} (5 alike) : Constant  Value=0.1  OutDataTypeStr=single
  Constant5 : Constant  Value=10  OutDataTypeStr=int16
  Constant6 : Constant  Value=20  OutDataTypeStr=int16
  Constant7 : Constant  Value=30  OutDataTypeStr=int16
  Constant8 : Constant  Value=40  OutDataTypeStr=int16
  Constant9 : Constant  Value=50  OutDataTypeStr=int16
  Data Type Conversion : DataTypeConversion  OutDataTypeStr=uint16  SaturateOnIntegerOverflow=off  RndMeth=Floor
  Data Type Conversion1 : DataTypeConversion  OutDataTypeStr=int16  SaturateOnIntegerOverflow=off  RndMeth=Floor
  Product{,1..9} (10 alike) : Product  OutDataTypeStr=single
  Subsystem1 : Subsystem
  Subsystem2 : Subsystem
  Subsystem3 : Subsystem
  Subsystem4 : Subsystem
  Subsystem5 : Subsystem
  XCP : Subsystem
  Flow2Rpm : Outport
  wires:
  Subsystem1/1(Out1) -> Product/2
  Product2/1 -> Product7/2
  [breakpoint2] -> 2-D Lookup Table5/2
  Product4/1 -> Product9/2
  Product9/1 -> Add7/5
  [breakpoint1] -> 2-D Lookup Table7/1
  Constant9/1 -> Add6/1
  [breakpoint1] -> 2-D Lookup Table9/1
  [breakpoint1] -> 2-D Lookup Table5/1
  [breakpoint1] -> 2-D Lookup Table6/1
  Product5/1 -> Add7/1
  2-D Lookup Table7/1 -> Product2/1
  Data Type Conversion1/1 -> Add4/2, Add6/2, Add5/2, Add3/2, Add2/2
  [breakpoint2] -> 2-D Lookup Table8/2
  Product/1 -> Product5/2
  Subsystem5/1(Out1) -> Product4/2
  [breakpoint2] -> 2-D Lookup Table7/2
  Subsystem2/1(Out1) -> Product1/2
  Constant8/1 -> Add5/1
  Product8/1 -> Add7/4
  Constant7/1 -> Add4/1
  Add4/1 -> Subsystem3/1(In1)
  Subsystem3/1(Out1) -> Product2/2
  Subsystem4/1(Out1) -> Product3/2
  Product1/1 -> Product6/2
  Add2/1 -> Subsystem1/1(In1)
  [breakpoint1] -> 2-D Lookup Table8/1
  [breakpoint2] -> 2-D Lookup Table6/2
  2-D Lookup Table5/1 -> Product/1
  Constant5/1 -> Add2/1
  2-D Lookup Table8/1 -> Product3/1
  Constant6/1 -> Add3/1
  Add6/1 -> Subsystem5/1(In1)
  Add5/1 -> Subsystem4/1(In1)
  Product3/1 -> Product8/2
  [breakpoint2] -> 2-D Lookup Table9/2
  Add3/1 -> Subsystem2/1(In1)
  Add7/1 -> Data Type Conversion/1
  2-D Lookup Table6/1 -> Product1/1
  Product7/1 -> Add7/3
  2-D Lookup Table9/1 -> Product4/1
  Product6/1 -> Add7/2
  breakpoint1/1 -> [breakpoint1]
  breakpoint2/1 -> [breakpoint2]
  XCP/1(Out1) -> Data Type Conversion1/1
  Constant/1 -> Product5/1
  Constant1/1 -> Product6/1
  Constant2/1 -> Product7/1
  Constant3/1 -> Product8/1
  Constant4/1 -> Product9/1
  md_u8Blw/1 -> XCP/1(md_u8Blw)
  Data Type Conversion/1 -> Flow2Rpm/1
